simulink model "sf_server"  (R2017b)
settings: Solver=ode45  StartTime=0.0  StopTime=inf  RelTol=1e-3  EnableMultiTasking=on
PreLoadFcn:
  | queueLength = 10;
CloseFcn:
  | delete(findall(0, 'type', 'figure', 'tag', 'SF_SERVER'))
  | clear('queueLength')
settings Model: ExtModeAutoUpdateStatusClock=off  Creator=The MathWorks, Inc.  LastModifiedBy=The MathWorks, Inc.
settings DataIOCC: LimitDataPoints=on  SaveFormat=Array  SignalLoggingName=logsOut
settings OptimizationCC: ExpressionDepthLimit=2147483647  InitFltsAndDblsToZero=on  EfficientMapNaN2IntZero=off  LifeSpan=inf
settings DebuggingCC: UnderspecifiedInitializationDetection=Classic  MergeDetectMultiDrivingBlocksExec=none  CheckExecutionContextPreStartOutputMsg=on  CheckExecutionContextRuntimeOutputMsg=on  SignalResolutionControl=TryResolveAllWithWarning  MultiTaskDSMMsg=warning  MultiTaskCondExecSysMsg=none  FcnCallInpInsideContextMsg=warning  StateNameClashWarn=warning  SFUnexpectedBacktrackingDiag=warning  SFNoUnconditionalDefaultTransitionDiag=warning  SFExecutionAtInitializationDiag=none  SFMachineParentedDataDiag=none
settings HardwareCC: ProdBitPerPointer=32  ProdBitPerSizeT=32  ProdBitPerPtrDiffT=32  ProdLargestAtomicFloat=None  ProdIntDivRoundTo=Undefined  ProdEndianess=Unspecified  ProdWordSize=32  ProdHWDeviceType=32-bit Generic  TargetUnknown=on
settings ModelReferenceCC: PropagateSignalLabelsOutOfModel=off
settings SFSimCC: SimParseCustomCode=off
settings CodeAppCC: StateflowObjectComments=on
settings GRTTargetCC: TargetLangStandard=C89/C90 (ANSI)  GeneratePreprocessorConditionals=Disable all  CombineOutputUpdateFcns=off  GRTInterface=on
settings ConfigComp: CovMetricSettings=dcmtr  CovHtmlReporting=on  CovSaveCumulativeToWorkspaceVar=on  CovSaveSingleToWorkspaceVar=on  CovExternalEMLEnable=off  CovSFcnEnable=off

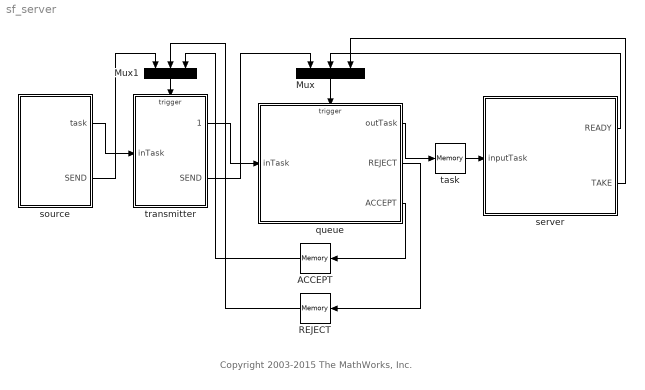
== system sf_server ==
  note: Copyright 2003-2015 The MathWorks, Inc.
  ACCEPT : Memory
  Mux : Mux  Inputs=3
  Mux1 : Mux  Inputs=3
  REJECT : Memory
  queue : Stateflow chart  TreatAsAtomicUnit=on
  server : Stateflow chart  TreatAsAtomicUnit=on
  source : Stateflow chart  TreatAsAtomicUnit=on
  task : Memory
  transmitter : Stateflow chart  TreatAsAtomicUnit=on
  wires:
  queue/1(outTask) -> task/1
  transmitter/1(outTask) -> queue/1(inTask)
  transmitter/2(SEND) -> Mux/1
  server/1(READY) -> Mux/2
  Mux/1 -> queue/Trigger
  server/2(TAKE) -> Mux/3
  source/1(task) -> transmitter/1(inTask)
  source/2(SEND) -> Mux1/1
  Mux1/1 -> transmitter/Trigger
  queue/2(REJECT) -> REJECT/1
  task/1 -> server/1(inputTask)
  REJECT/1 -> Mux1/2
  queue/3(ACCEPT) -> ACCEPT/1
  ACCEPT/1 -> Mux1/3

== stateflow chart sf_server/queue ==
  state Queue [group]
    state b = is_empty() [function]
      (default) -> (junction 26) : {b = front == back && !incremented;}
    state b = is_full() [function]
      (default) -> (junction 34) : {b = front == back && incremented;}
    state next = increment(i) [function]
      (default) -> (junction 33) : {next = i+1;}
      (junction 33) -> (junction 27) : [next > queueLength]
          | {next = 1;}
    state enqueue(d) [function]
      (default) -> (junction 28)
      (junction 28) -> (junction 29) [order 1] : [is_full()]
          | {ml.error('Queue overflow');}
      (junction 28) -> (junction 30) [order 2] : {back = increment(back);
          | incremented = 1;
          | data[back] = d;
          | set_queue(data, front, back, is_full());}
    state d = dequeue() [function]
      (default) -> (junction 31)
      (junction 31) -> (junction 32) [order 1] : [is_empty()]
          | {ml.error('Queue underflow');}
      (junction 31) -> (junction 35) [order 2] : {front = increment(front);
          | incremented = 0;
          | d = data[front];
          | set_queue(data, front, back, 0);}
  (default) -> (junction 25) [order 1] : ENQUEUE
  (junction 25) -> (junction 37) [order 1] : [Queue.is_full()]
      | {REJECT;}
  (junction 25) -> (junction 38) [order 2] : {ACCEPT;
      | Queue.enqueue(inTask);}
  (default) -> (junction 41) [order 2] : DEQUEUE
  (junction 41) -> (junction 40) [order 1] : [Queue.is_empty()]
      | {outTask = 0;}
  (junction 41) -> (junction 39) [order 2] : {outTask = Queue.dequeue();}
  (default) -> (junction 36) [order 3] : CLEAR
      | {outTask = 0;}
  data: b function_output boolean size=1; b function_output boolean size=1; next function_output int32 size=1; i function_input int32 size=1; d function_input int32 size=1; d function_output int32 size=1; data local double size=queueLength; front local double size=1; back local double size=1; incremented local boolean size=1; queue function_input double size=queueLength; front function_input double size=1; back function_input double size=1; isFull function_input double size=1; inTask input double size=1; outTask output double size=1
  events: ENQUEUE input EITHER_EDGE_EVENT; DEQUEUE input EITHER_EDGE_EVENT; CLEAR input EITHER_EDGE_EVENT; REJECT output EITHER_EDGE_EVENT; ACCEPT output EITHER_EDGE_EVENT
  function set_queue(queue, front, back, isFull):
    | function set_queue(queue, front, back, isFull)
    | 
    |     coder.extrinsic('int2str', 'set', 'sf_server_handle_map');
    |     
    |     for i = queueLength:-1:1
    | 
    |         if front ~= back || isFull
    |             front = increment(front);
    |             isFull = 0;
    |             set(sf_server_handle_map('queueText', i), 'String', int2str(queue(front)));
    |         else
    |             set(sf_server_handle_map('queueText', i), 'String', '');
    |         end        
    |     end
    | 
    | function i = increment(i)
    |     i = i + 1;
    |     if i > queueLength
    |         i = 1;
    |     end

== stateflow chart sf_server/server ==
  state Idle
    READY;
  state Busy
  Idle -> Idle [order 2]
  (default) -> Idle
  Idle -> Busy [order 1] : [inputTask]
      | {taskTime = 2*inputTask;
      | TAKE;
      | process_task(inputTask);}
  Busy -> Idle : [after(taskTime, tick)]
      | {process_task(0);}
  data: task function_input double size=1; inputTask input double size=1; taskTime local double size=1
  events: READY output EITHER_EDGE_EVENT; TAKE output EITHER_EDGE_EVENT
  function process_task(task):
    | function process_task(task)
    | 
    | coder.extrinsic('int2str', 'set', 'sf_server_handle_map');
    | processText = sf_server_handle_map('processText');
    | string = ' ';
    | 
    | if task
    |     string = int2str(task);
    | end
    | 
    | set(processText, 'String', string);

== stateflow chart sf_server/transmitter ==
  (default) -> (junction 8) [order 1] : TRANSMIT
      | {send_task(inTask);
      | outTask = inTask;
      | SEND;}
  (default) -> (junction 9) [order 2] : REJECT
      | {reject_task();}
  (default) -> (junction 10) [order 3] : ACCEPT
      | {accept_task();}
  data: task function_input double size=1; outTask output double size=1; inTask input double size=1
  events: SEND output EITHER_EDGE_EVENT; TRANSMIT input EITHER_EDGE_EVENT; REJECT input EITHER_EDGE_EVENT; ACCEPT input EITHER_EDGE_EVENT
  function init_gui:
    | function init_gui
    | 
    | coder.extrinsic('set', 'findall', 'figure', 'delete', 'axes', 'text', 'rectangle', 'sf_server_handle_map', 'is_invalid_gui_obj_handle');
    | fig = sf_server_handle_map('fig');
    | 
    | if is_invalid_gui_obj_handle(fig)
    |     % see if there is an existing figure
    |     figTemp = findall(0, 'type', 'figure', 'tag', 'SF_SERVER');
    |     if ~isempty(figTemp)
    |         deleteFig = 0;
    |         
    |         fig = figTemp;
    |         lastObj = fig;
    |         sf_server_handle_map('fig', fig);
    |         
    |         sendText = feval('get', lastObj, 'UserData');
    |         lastObj = sendText;
    |         sf_server_handle_map('sendText', sendText);
    |         
    |         for i = 1:queueLength
    |             queueItemText = feval('get', lastObj, 'UserData');
    | 
    |             if ~queueItemText
    |                 deleteFig = 1;
    |                 break;
    |             end
    |             
    |             sf_server_handle_map(i, queueItemText);
    |             
    |             set(queueItemText, 'String', '');
    |             lastObj = queueItemText;
    |         end
    |         
    |         if ~deleteFig
    |             processText = feval('get', lastObj, 'UserData');
    |             if ~processText
    |                 deleteFig = 1;
    |             else
    |                 deleteFig = feval('get', processText, 'UserData');
    |             end
    |             sf_server_handle_map('processText', processText);
    |         end
    |         if deleteFig
    |             delete(fig);
    |             fig = 0;
    |         end
    |     end
    | end
    | 
    | if is_invalid_gui_obj_handle(fig)
    |     % screen size etiqette
    |     units = 'points';
    |     screenUnits = feval('get', 0, 'Units');
    |     set(0, 'Units', units);
    |     screenSize = zeros(1,4);
    |     screenSize = feval('get', 0, 'ScreenSize');
    |     set(0, 'Units', screenUnits);
    |     
    |     backgroundColor = feval('get', 0, 'DefaultUIControlBackgroundColor');
    | 
    |     fontSize = 48;
    |     buffer = 10;
    |     textWidth = 35;    
    |     textY = 50;
    |     rectHeight = 60;
    |     rectWidth = textWidth-5;
    |     rectY = textY - rectHeight/2;
    | 
    |     
    |     % default figure size
    |     figureHeight = 2*textY;
    |     figureWidth = 4*buffer+(queueLength+2)*textWidth;
    | 
    |     % make sure the initial size is less than 90% of the screen in either direction
    |     figureWidth = min(figureWidth, .9*screenSize(3));
    |     figureHeight = min(figureHeight, .9*screenSize(4));
    | 
    |     fig = figure('doubleBuffer', 'on',...
    |                  'MenuBar', 'none',...
    |                  'Name', 'Server Display',...
    |                  'Tag', 'SF_SERVER',...
    |                  'NumberTitle', 'off',...
    |                  'HandleVisibility', 'off',...
    |                  'IntegerHandle', 'off',...
    |                  'Color', backgroundColor,...
    |                  'Units', units,...
    |                  'DefaultUIControlUnits', units,...
    |                  'Position', [(screenSize(3)-figureWidth)/2 (screenSize(4)-figureHeight)/2 figureWidth figureHeight]);
    |              
    |     sf_server_handle_map('fig', fig);
    | 
    |     lastObj = fig;
    |     
    |     figAxes = axes('Parent', fig,...
    |                    'Visible', 'off',...
    |                    'Position', [0 0 1 1],...
    |                    'XLim', [0 figureWidth],...
    |                    'YLim', [0 figureHeight]);
    | 
    |     sendText = text(buffer, textY, '',...
    |                     'Parent', figAxes,...
    |                     'Color', 'blue',...
    |                     'BackgroundColor', backgroundColor,...
    |                     'FontSize', fontSize);
    |                 
    |     sf_server_handle_map('sendText', sendText);
    | 
    |     set(lastObj, 'UserData', sendText);
    |     lastObj = sendText;
    |     
    |     for i = 1:queueLength
    |         rectangle('Position', [2*buffer+i*textWidth-2, rectY, rectWidth, rectHeight],...
    |                   'FaceColor', 'black',...
    |                   'EdgeColor', 'none',...
    |                   'Parent', figAxes);
    |         queueItemText = text(2*buffer+i*textWidth, textY, '',...
    |                             'Parent', figAxes,...
    |                             'Color', 'green',...
    |                             'BackgroundColor', 'black',...
    |                             'FontSize', fontSize);
    |         set(lastObj, 'UserData', queueItemText);
    |         lastObj = queueItemText;
    |         sf_server_handle_map('queueText', i, queueItemText);
    |     end
    |    
    |     processText = text(3*buffer+(queueLength+1)*textWidth, textY, '',...
    |                        'Parent', figAxes,...
    |                        'Color', 'black',...
    |                        'BackgroundColor', backgroundColor,...
    |                        'FontSize', fontSize,...
    |                        'UserData', 0);
    |     sf_server_handle_map('processText', processText);
    |     set(lastObj, 'UserData', processText);
    | end
  function send_task(task):
    | function send_task(task)
    | coder.extrinsic('set', 'ishandle', 'int2str', 'sf_server_handle_map', 'is_invalid_gui_obj_handle');
    | fig = sf_server_handle_map('fig');
    | if is_invalid_gui_obj_handle(fig)
    |     init_gui;    
    | end
    | sendText = sf_server_handle_map('sendText');
    | set(sendText, 'String', int2str(task), 'Color', 'blue');
  function reject_task:
    | function reject_task
    | coder.extrinsic('set', 'ishandle', 'sf_server_handle_map', 'is_invalid_gui_obj_handle');
    | fig = sf_server_handle_map('fig');
    | if is_invalid_gui_obj_handle(fig)
    |     init_gui;
    | end
    | sendText = sf_server_handle_map('sendText');
    | set(sendText, 'Color', 'red');
  function accept_task:
    | function accept_task
    | coder.extrinsic('set', 'ishandle', 'sf_server_handle_map', 'is_invalid_gui_obj_handle');
    | fig = sf_server_handle_map('fig');
    | if is_invalid_gui_obj_handle(fig)
    |     init_gui;
    | end
    | sendText = sf_server_handle_map('sendText');
    | set(sendText, 'String', '');

== stateflow chart sf_server/source ==
  state Send
  state Pause
    ex: ml.pause(.1);
  (default) -> Send
  Pause -> Send
  Send -> (junction 24) : {x = ml.floor(ml.rand()*20);}
  (junction 36) -> Pause
  (junction 24) -> (junction 25) [order 1] : [x>=19]{task = 5;}
  (junction 25) -> (junction 27)
  (junction 24) -> (junction 26) [order 2]
  (junction 26) -> (junction 27) [order 1] : [x>=18]{task = 4;}
  (junction 26) -> (junction 28) [order 2]
  (junction 27) -> (junction 29)
  (junction 28) -> (junction 29) [order 1] : [x>=17]{task = 3;}
  (junction 28) -> (junction 30) [order 2]
  (junction 29) -> (junction 31)
  (junction 30) -> (junction 31) [order 1] : [x>=15]{task = 2;}
  (junction 30) -> (junction 32) [order 2]
  (junction 31) -> (junction 33)
  (junction 32) -> (junction 33) [order 1] : [x>=14]{task = 1;}
  (junction 32) -> (junction 35) [order 2]
  (junction 33) -> (junction 34) : {SEND;}
  (junction 35) -> (junction 34)
  (junction 34) -> (junction 36)
  data: x local double size=1; task output double size=1
  events: SEND output EITHER_EDGE_EVENT
